simulink model "ICN_with_BR_input_model4test_clusterParams_ICNtune_v13_RSA_25Hz"  (R2020b)
settings: Solver=ode15s  StartTime=0.5  StopTime=300  RelTol=1e-3  EnableMultiTasking=on
model workspace (MAT data in the model file):
  HRResponseIano = [1 0.976355617701 1.05061592575 1.14391807051 1.22959062218 1.30026078221 1.35513299833 1.39551709306 1.423380234 1.44057518669 1.44870724956 1.44945189675 ... (1201 elements, 1x1201)]
values from neighbouring files (symbols this model uses):
  LBNP_input = Simulink.Parameter(LBNP_input)    [BRclosedLoop_model_initialize_params.m]
libraries: simulink x1
(part 1 of 2)
settings Model: OrderedModelArguments=off  Creator=parkjams  LastModifiedBy=mmgee
settings SolverCC: ZeroCrossAlgorithm=Adaptive
settings DataIOCC: SaveFormat=StructureWithTime  ReturnWorkspaceOutputs=off
settings OptimizationCC: LifeSpan=inf
settings DebuggingCC: IgnoredZcDiagnostic=none  SFUnexpectedBacktrackingDiag=warning  SFNoUnconditionalDefaultTransitionDiag=warning  SFExecutionAtInitializationDiag=none  ArithmeticOperatorsInVariantConditions=warning
settings HardwareCC: ProdBitPerSizeT=32  ProdBitPerPtrDiffT=32  ProdWordSize=32  ProdHWDeviceType=Specified  TargetBitPerPointer=64  TargetBitPerSizeT=64  TargetBitPerPtrDiffT=64  TargetLongLongMode=on  TargetIntDivRoundTo=Zero  TargetEndianess=LittleEndian  TargetWordSize=64  TargetHWDeviceType=MATLAB Host  ProdEqTarget=off
settings ModelReferenceCC: PropagateSignalLabelsOutOfModel=off
settings SFSimCC: SimUseLocalCustomCode=off  CustomCodeUndefinedFunction=UseInterfaceOnly
settings RTWCC: Description=Rapid Simulation Target  SystemTargetFile=rsim.tlc  TemplateMakefile=rsim_default_tmf  RTWUseLocalCustomCode=off
settings CodeAppCC: StateflowObjectComments=on
settings ConfigComp: CovMetricSettings=dw  CovSaveCumulativeToWorkspaceVar=on  CovSaveSingleToWorkspaceVar=on  CovExternalEMLEnable=off

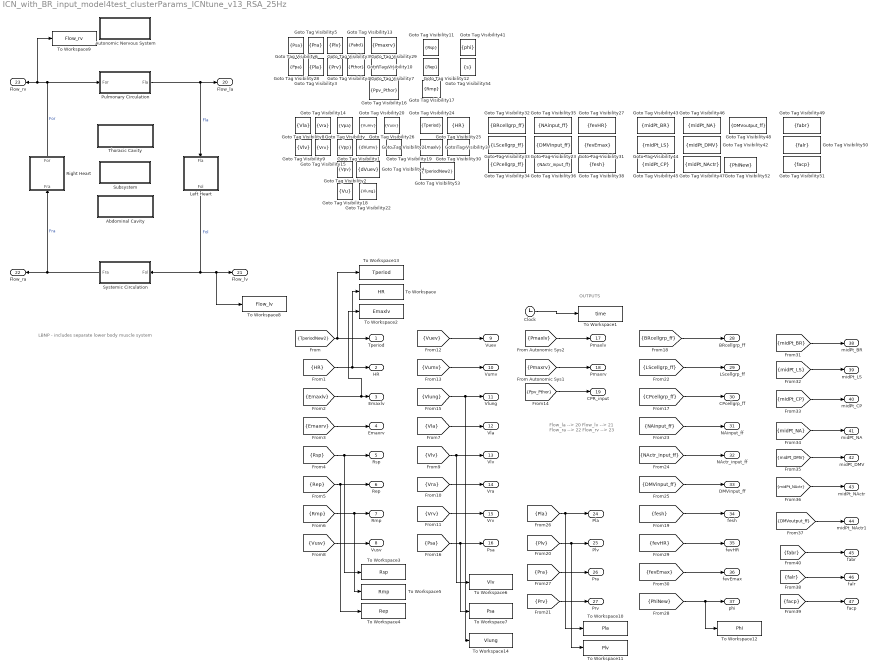
== system ICN_with_BR_input_model4test_clusterParams_ICNtune_v13_RSA_25Hz ==
  note: Flow_la --> 20
      |
      | Flow_lv --> 21
      |
      | Flow_ra --> 22
      |
      | Flow_rv --> 23
  note: OUTPUTS
  note: LBNP - includes separate lower body muscle system
  Abdominal Cavity : Subsystem
      mask Display: disp('Abdominal Cavity')
  Autonomic Nervous System : Subsystem
      mask Display: disp('Autonomic \n Nervous System')
  Clock : Clock
  Goto Tag Visibility : GotoTagVisibility  GotoTag=Vpa
  Goto Tag Visibility1 : GotoTagVisibility  GotoTag=Vpp
  Goto Tag Visibility10 : GotoTagVisibility  GotoTag=Pthor
  Goto Tag Visibility11 : GotoTagVisibility  GotoTag=Rsp
  Goto Tag Visibility12 : GotoTagVisibility  GotoTag=Rep
  Goto Tag Visibility13 : GotoTagVisibility  GotoTag=Pabd
  Goto Tag Visibility14 : GotoTagVisibility  GotoTag=Vra
  Goto Tag Visibility15 : GotoTagVisibility  GotoTag=Vrv
  Goto Tag Visibility16 : GotoTagVisibility  GotoTag=Ppv_Pthor
  Goto Tag Visibility17 : GotoTagVisibility  GotoTag=Rmp
  Goto Tag Visibility18 : GotoTagVisibility  GotoTag=Vu
  Goto Tag Visibility19 : GotoTagVisibility  GotoTag=Vuev
  Goto Tag Visibility2 : GotoTagVisibility  GotoTag=Vpv
  Goto Tag Visibility20 : GotoTagVisibility  GotoTag=Vumv
  Goto Tag Visibility21 : GotoTagVisibility  GotoTag=dVumv
  Goto Tag Visibility22 : GotoTagVisibility  GotoTag=Vlung
  Goto Tag Visibility23 : GotoTagVisibility  GotoTag=DMVinput_ff
  Goto Tag Visibility24 : GotoTagVisibility  GotoTag=Tperiod
  Goto Tag Visibility25 : GotoTagVisibility  GotoTag=HR
  Goto Tag Visibility26 : GotoTagVisibility  GotoTag=Vusv
  Goto Tag Visibility27 : GotoTagVisibility  GotoTag=fevHR
  Goto Tag Visibility28 : GotoTagVisibility  GotoTag=Ppa
  Goto Tag Visibility29 : GotoTagVisibility  GotoTag=Pmaxrv
  Goto Tag Visibility3 : GotoTagVisibility  GotoTag=Pla
  Goto Tag Visibility30 : GotoTagVisibility  GotoTag=Emaxrv
  Goto Tag Visibility31 : GotoTagVisibility  GotoTag=fevEmax
  Goto Tag Visibility32 : GotoTagVisibility  GotoTag=BRcellgrp_ff
  Goto Tag Visibility33 : GotoTagVisibility  GotoTag=LScellgrp_ff
  Goto Tag Visibility34 : GotoTagVisibility  GotoTag=CPcellgrp_ff
  Goto Tag Visibility35 : GotoTagVisibility  GotoTag=NAinput_ff
  Goto Tag Visibility36 : GotoTagVisibility  GotoTag=NActr_input_ff
  Goto Tag Visibility37 : GotoTagVisibility  GotoTag=Emaxlv
  Goto Tag Visibility38 : GotoTagVisibility  GotoTag=fesh
  Goto Tag Visibility39 : GotoTagVisibility  GotoTag=Plv
  Goto Tag Visibility4 : GotoTagVisibility  GotoTag=dVuev
  Goto Tag Visibility40 : GotoTagVisibility  GotoTag=Prv
  Goto Tag Visibility41 : GotoTagVisibility  GotoTag=phi
  Goto Tag Visibility42 : GotoTagVisibility  GotoTag=midPt_DMV
  Goto Tag Visibility43 : GotoTagVisibility  GotoTag=midPt_BR
  Goto Tag Visibility44 : GotoTagVisibility  GotoTag=midPt_LS
  Goto Tag Visibility45 : GotoTagVisibility  GotoTag=midPt_CP
  Goto Tag Visibility46 : GotoTagVisibility  GotoTag=midPt_NA
  Goto Tag Visibility47 : GotoTagVisibility  GotoTag=midPt_NActr
  Goto Tag Visibility48 : GotoTagVisibility  GotoTag=DMVoutput_ff
  Goto Tag Visibility49 : GotoTagVisibility  GotoTag=fabr
  Goto Tag Visibility5 : GotoTagVisibility  GotoTag=Pra
  Goto Tag Visibility50 : GotoTagVisibility  GotoTag=falr
  Goto Tag Visibility51 : GotoTagVisibility  GotoTag=facp
  Goto Tag Visibility52 : GotoTagVisibility  GotoTag=PhiNew
  Goto Tag Visibility53 : GotoTagVisibility  GotoTag=TperiodNew2
  Goto Tag Visibility54 : GotoTagVisibility  GotoTag=s
  Goto Tag Visibility6 : GotoTagVisibility  GotoTag=Psa
  Goto Tag Visibility7 : GotoTagVisibility  GotoTag=Pmaxlv
  Goto Tag Visibility8 : GotoTagVisibility  GotoTag=Vla
  Goto Tag Visibility9 : GotoTagVisibility  GotoTag=Vlv
  Left Heart : Subsystem
      mask Display: disp('Left Heart')
  Pulmonary Circulation : Subsystem
      mask Display: disp('Pulmonary \n Circulation')
  Right Heart : Subsystem
      mask Display: disp('Right Heart')
  Subsystem : Subsystem
      mask Display: disp('Lungs')
  Systemic Circulation : Subsystem
      mask Display: disp('Systemic \n Circulation')
  Thoracic Cavity : Subsystem
      mask Display: disp('Thoracic Cavity')
  To Workspace : ToWorkspace  VariableName=HR  SampleTime=-1
  To Workspace1 : ToWorkspace  VariableName=time  SampleTime=-1
  To Workspace10 : ToWorkspace  VariableName=Pla  SampleTime=-1
  To Workspace11 : ToWorkspace  VariableName=Plv  SampleTime=-1
  To Workspace12 : ToWorkspace  VariableName=Phi  SampleTime=-1
  To Workspace13 : ToWorkspace  VariableName=Tperiod  SampleTime=-1
  To Workspace14 : ToWorkspace  VariableName=Vlung  SampleTime=-1
  To Workspace2 : ToWorkspace  VariableName=Emaxlv  SampleTime=-1
  To Workspace3 : ToWorkspace  VariableName=Rsp  SaveFormat=Timeseries  SampleTime=-1
  To Workspace4 : ToWorkspace  VariableName=Rep  SaveFormat=Timeseries  SampleTime=-1
  To Workspace5 : ToWorkspace  VariableName=Rmp  SaveFormat=Timeseries  SampleTime=-1
  To Workspace6 : ToWorkspace  VariableName=Vlv  SampleTime=-1
  To Workspace7 : ToWorkspace  VariableName=Psa  SampleTime=-1
  To Workspace8 : ToWorkspace  VariableName=Flow_lv  SampleTime=-1
  To Workspace9 : ToWorkspace  VariableName=Flow_rv  SampleTime=-1
  Tperiod : Outport
  HR : Outport  Port=2
  Emaxlv : Outport  Port=3
  Emaxrv : Outport  Port=4
  Rsp : Outport  Port=5
  Rep : Outport  Port=6
  Rmp : Outport  Port=7
  Vusv : Outport  Port=8
  Vuev : Outport  Port=9
  Vumv : Outport  Port=10
  Vlung : Outport  Port=11
  Vla : Outport  Port=12
  Vlv : Outport  Port=13
  Vra : Outport  Port=14
  Vrv : Outport  Port=15
  Psa : Outport  Port=16
  Pmaxlv : Outport  Port=17
  Pmaxrv : Outport  Port=18
  CPR_input : Outport  Port=19
  Flow_la : Outport  Port=20
  Flow_lv : Outport  Port=21
  Flow_ra : Outport  Port=22
  Flow_rv : Outport  Port=23
  Pla : Outport  Port=24
  Plv : Outport  Port=25
  Pra : Outport  Port=26
  Prv : Outport  Port=27
  BRcellgrp_ff : Outport  Port=28
  LScellgrp_ff : Outport  Port=29
  CPcellgrp_ff : Outport  Port=30
  NAinput_ff : Outport  Port=31
  NActr_input_ff : Outport  Port=32
  DMVinput_ff : Outport  Port=33
  fesh : Outport  Port=34
  fevHR : Outport  Port=35
  fevEmax : Outport  Port=36
  phi : Outport  Port=37
  midPt_BR : Outport  Port=38
  midPt_LS : Outport  Port=39
  midPt_CP : Outport  Port=40
  midPt_NA : Outport  Port=41
  midPt_DMV : Outport  Port=42
  midPt_NActr : Outport  Port=43
  midPt_NActr1 : Outport  Port=44
  fabr : Outport  Port=45
  falr : Outport  Port=46
  facp : Outport  Port=47
  wires:
  Pulmonary Circulation/1(Fla) -> Left Heart/1(Fla), Flow_la/1  "Fla"
  Right Heart/1(For) -> To Workspace9/1, Flow_rv/1, Pulmonary Circulation/1(For)  "For"
  Left Heart/1(Fol) -> Systemic Circulation/1(Fol), To Workspace8/1, Flow_lv/1  "Fol"
  Systemic Circulation/1(Fra) -> Right Heart/1(Fra), Flow_ra/1  "Fra"
  [TperiodNew2] -> To Workspace13/1, Tperiod/1
  [HR] -> To Workspace/1, HR/1
  [Emaxlv] -> To Workspace2/1, Emaxlv/1
  [Emaxrv] -> Emaxrv/1
  [Rsp] -> To Workspace3/1, Rsp/1
  [Rep] -> To Workspace4/1, Rep/1
  [Rmp] -> To Workspace5/1, Rmp/1
  [Vusv] -> Vusv/1
  [Vuev] -> Vuev/1
  [Vumv] -> Vumv/1
  [Vlung] -> To Workspace14/1, Vlung/1
  [Vla] -> Vla/1
  [Vlv] -> To Workspace6/1, Vlv/1
  [Vra] -> Vra/1
  [Vrv] -> Vrv/1
  [Psa] -> To Workspace7/1, Psa/1
  [Pmaxlv] -> Pmaxlv/1
  [Pmaxrv] -> Pmaxrv/1
  [Ppv_Pthor] -> CPR_input/1
  [Pla] -> To Workspace10/1, Pla/1
  [Plv] -> To Workspace11/1, Plv/1
  [Pra] -> Pra/1
  [Prv] -> Prv/1
  [BRcellgrp_ff] -> BRcellgrp_ff/1
  [LScellgrp_ff] -> LScellgrp_ff/1
  [CPcellgrp_ff] -> CPcellgrp_ff/1
  [NAinput_ff] -> NAinput_ff/1
  [NActr_input_ff] -> NActr_input_ff/1
  [DMVinput_ff] -> DMVinput_ff/1
  [fesh] -> fesh/1
  [fevHR] -> fevHR/1
  [fevEmax] -> fevEmax/1
  [PhiNew] -> To Workspace12/1, phi/1
  [midPt_BR] -> midPt_BR/1
  [midPt_LS] -> midPt_LS/1
  [midPt_CP] -> midPt_CP/1
  [midPt_NA] -> midPt_NA/1
  [midPt_DMV] -> midPt_DMV/1
  [midPt_NActr] -> midPt_NActr/1
  [DMVoutput_ff] -> midPt_NActr1/1
  [fabr] -> fabr/1
  [falr] -> falr/1
  [facp] -> facp/1
  Clock/1 -> To Workspace1/1

== system ICN_with_BR_input_model4test_clusterParams_ICNtune_v13_RSA_25Hz/Abdominal Cavity ==
  (Tinsp + Texp)/Tresp : Switch  Criteria=u2 > Threshold  Threshold=(1.6 + 1.4)/4
  Abdominal condition 1 : Subsystem
  Abdominal condition 2 : Subsystem
  Constant : Constant  Value=-2.5
  Constant2 : Constant  Value=0
  Integral threshold : Constant
  Integrator3 : Integrator  ExternalReset=falling  ShowStatePort=on
  Math Function3 : Math  Operator=reciprocal  SignedPower=on  SaturateOnIntegerOverflow=on
  Sum3 : Sum  Inputs=-+
  Tinsp/(2*Tresp) : Switch  Criteria=u2 > Threshold  Threshold=1.6/(2*4)
  Tinsp/Tresp : Switch  Criteria=u2 > Threshold  Threshold=1.6/4
  Tresp : Constant  Value=4
  tag scope: Pabd=scoped
  wires:
  Tresp/1 -> Math Function3/1
  Math Function3/1 -> Integrator3/1
  Integrator3/State -> Sum3/1
  Integral threshold/1 -> Sum3/2
  Sum3/1 -> Integrator3/2
  Integrator3/1 -> Abdominal condition 1/1(S (resp)), (Tinsp + Texp)/Tresp/2, Abdominal condition 2/1(S (resp)), Tinsp/Tresp/2, Tinsp/(2*Tresp)/2
  Abdominal condition 1/1(Out1) -> Tinsp/(2*Tresp)/3
  Constant/1 -> Tinsp/(2*Tresp)/1
  Tinsp/(2*Tresp)/1 -> Tinsp/Tresp/3
  Abdominal condition 2/1(Out1) -> Tinsp/Tresp/1
  Tinsp/Tresp/1 -> (Tinsp + Texp)/Tresp/3
  Constant2/1 -> (Tinsp + Texp)/Tresp/1
  (Tinsp + Texp)/Tresp/1 -> [Pabd]

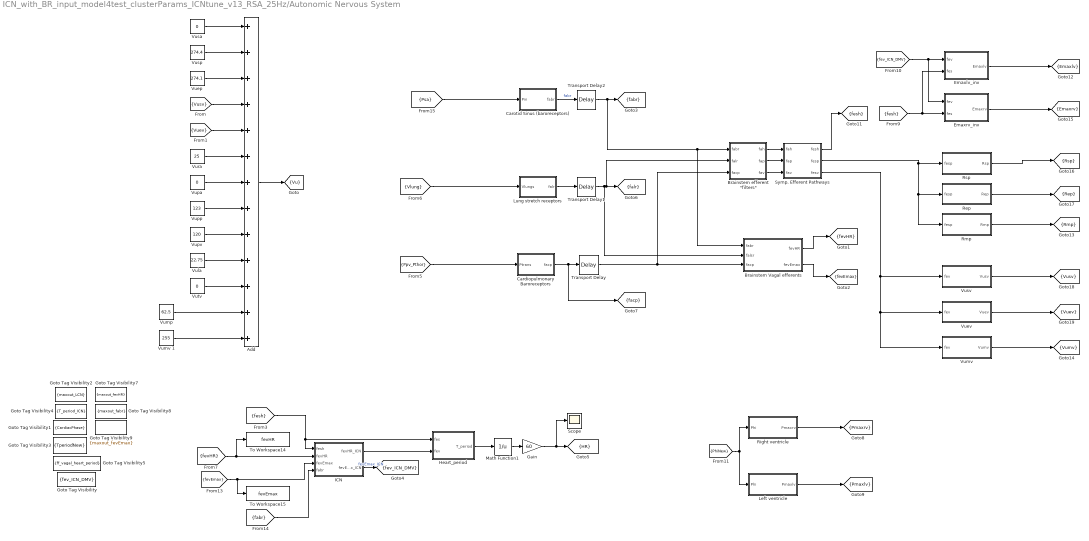
== system ICN_with_BR_input_model4test_clusterParams_ICNtune_v13_RSA_25Hz/Autonomic Nervous System ==
  " Brainstem efferent \"filters\"" : Subsystem
  " Symp. Efferent Pathways" : Subsystem
  Add : Sum  Inputs=+++++++++++++
  "Brainstem Vagal efferents " : Subsystem
  Cardiopulmonary Baroreceptors : Subsystem
  Carotid Sinus (baroreceptors) : Subsystem
  Emaxlv_inv : Subsystem
  Emaxrv_inv : Subsystem
  Gain : Gain  Gain=60
  Goto Tag Visibility : GotoTagVisibility  GotoTag=fev_ICN_DMV
  Goto Tag Visibility1 : GotoTagVisibility  GotoTag=CardiacPhase
  Goto Tag Visibility2 : GotoTagVisibility  GotoTag=maxout_LCN
  Goto Tag Visibility3 : GotoTagVisibility  GotoTag=TperiodNew
  Goto Tag Visibility4 : GotoTagVisibility  GotoTag=T_period_ICN
  Goto Tag Visibility5 : GotoTagVisibility  GotoTag=ff_vagal_heart_period
  Goto Tag Visibility7 : GotoTagVisibility  GotoTag=maxout_fevHR
  Goto Tag Visibility8 : GotoTagVisibility  GotoTag=maxout_fabr
  Goto Tag Visibility9 : GotoTagVisibility  GotoTag=maxout_fevEmax
  Heart_period : Subsystem
  ICN : Subsystem
  Left ventricle : Subsystem
  Lung stretch receptors : Subsystem
  Math Function1 : Math  Operator=reciprocal  SignedPower=on  SaturateOnIntegerOverflow=on
  Rep : Subsystem
  Right ventricle : Subsystem
  Rmp : Subsystem
  Rsp : Subsystem
  Scope : Scope
  To Workspace14 : ToWorkspace  VariableName=fevHR  SampleTime=-1
  To Workspace15 : ToWorkspace  VariableName=fevEmax  SampleTime=-1
  Transport Delay : TransportDelay  DelayTime=0.03
  Transport Delay1 : TransportDelay  DelayTime=0.03
  Transport Delay2 : TransportDelay  DelayTime=0.03
  Vuep : Constant  Value=274.1
  Vuev : Subsystem
  Vula : Constant  Value=22.75
  Vump : Constant  Value=62.5
  Vumv : Subsystem
  Vumv 1 : Constant  Value=255
  Vupa : Constant  Value=0
  Vupp : Constant  Value=123
  Vupv : Constant  Value=120
  Vura : Constant  Value=25
  Vusa : Constant  Value=0
  Vusp : Constant  Value=274.4
  Vusv : Subsystem
  Vutv : Constant  Value=0
  tag scope: Emaxlv=scoped, Emaxrv=scoped, HR=scoped, Pmaxlv=scoped, Pmaxrv=scoped, Rep=scoped, Rmp=scoped, Rsp=scoped, Vu=scoped, Vuev=scoped, Vumv=scoped, Vusv=scoped, fabr=scoped, facp=scoped, falr=scoped, fesh=scoped, fevEmax=scoped, fevHR=scoped, fev_ICN_DMV=scoped
  wires:
  Vusa/1 -> Add/1
  Vusp/1 -> Add/2
  [Vusv] -> Add/4
  [Vuev] -> Add/5
  Vuep/1 -> Add/3
  Vura/1 -> Add/6
  Vupa/1 -> Add/7
  Vupp/1 -> Add/8
  Vupv/1 -> Add/9
  Vula/1 -> Add/10
  Add/1 -> [Vu]
  Carotid Sinus (baroreceptors)/1(fabr) -> Transport Delay2/1  "fabr"
  Right ventricle/1(Pmaxrv) -> [Pmaxrv]
  Left ventricle/1(Pmaxlv) -> [Pmaxlv]
  Gain/1 -> Scope/1, [HR]
  Math Function1/1 -> Gain/1
  Rsp/1(Rsp) -> [Rsp]
  Rep/1(Rep) -> [Rep]
  Vusv/1(Vusv) -> [Vusv]
  Vuev/1(Vuev) -> [Vuev]
  Vumv/1(Vumv) -> [Vumv]
  Rmp/1(Rmp) -> [Rmp]
  Vump/1 -> Add/12
  Vumv 1/1 -> Add/13
  Lung stretch receptors/1(falr) -> Transport Delay1/1
  Vutv/1 -> Add/11
  [fesh] -> Emaxrv_inv/2(fes), Emaxlv_inv/2(fes)
  "Brainstem Vagal efferents "/2(fevEmax) -> [fevEmax]
  "Brainstem Vagal efferents "/1(fevHR) -> [fevHR]
  Emaxlv_inv/1(Emaxlv) -> [Emaxlv]
  Emaxrv_inv/1(Emaxrv) -> [Emaxrv]
  Cardiopulmonary Baroreceptors/1(facp) -> Transport Delay/1, [facp]
  " Brainstem efferent \"filters\""/1(fah) -> " Symp. Efferent Pathways"/1(fah)
  " Brainstem efferent \"filters\""/2(fap) -> " Symp. Efferent Pathways"/2(fap)
  " Symp. Efferent Pathways"/1(fesh) -> [fesh]
  " Symp. Efferent Pathways"/2(fesp) -> Rmp/1(fesp), Rep/1(fesp), Rsp/1(fesp)
  " Brainstem efferent \"filters\""/3(fav) -> " Symp. Efferent Pathways"/3(fav)
  " Symp. Efferent Pathways"/3(fesv) -> Vumv/1(fev), Vuev/1(fev), Vusv/1(fev)
  [fev_ICN_DMV] -> Emaxrv_inv/1(fev), Emaxlv_inv/1(fev)
  ICN/1(fevHR_ICN) -> Heart_period/2(fev)
  [PhiNew] -> Left ventricle/1(Phi), Right ventricle/1(Phi)
  Heart_period/1(T_period) -> Math Function1/1
  [fesh] -> ICN/1(fesh), Heart_period/1(fes)
  [fevEmax] -> ICN/3(fevEmax), To Workspace15/1
  [fabr] -> ICN/4(fabr)
  [fevHR] -> ICN/2(fevHR), To Workspace14/1
  [Vlung] -> Lung stretch receptors/1(Vlungs)
  [Psa] -> Carotid Sinus (baroreceptors)/1(Pin)
  Transport Delay/1 -> " Brainstem efferent \"filters\""/3(facp), "Brainstem Vagal efferents "/3(facp)
  Transport Delay1/1 -> "Brainstem Vagal efferents "/2(falsr), [falr], " Brainstem efferent \"filters\""/2(falr)
  Transport Delay2/1 -> "Brainstem Vagal efferents "/1(fabr), " Brainstem efferent \"filters\""/1(fabr), [fabr]
  [Ppv_Pthor] -> Cardiopulmonary Baroreceptors/1(Ptrans)
  ICN/2(fevEmax_ICN) -> [fev_ICN_DMV]  "fevEmax_ICN"

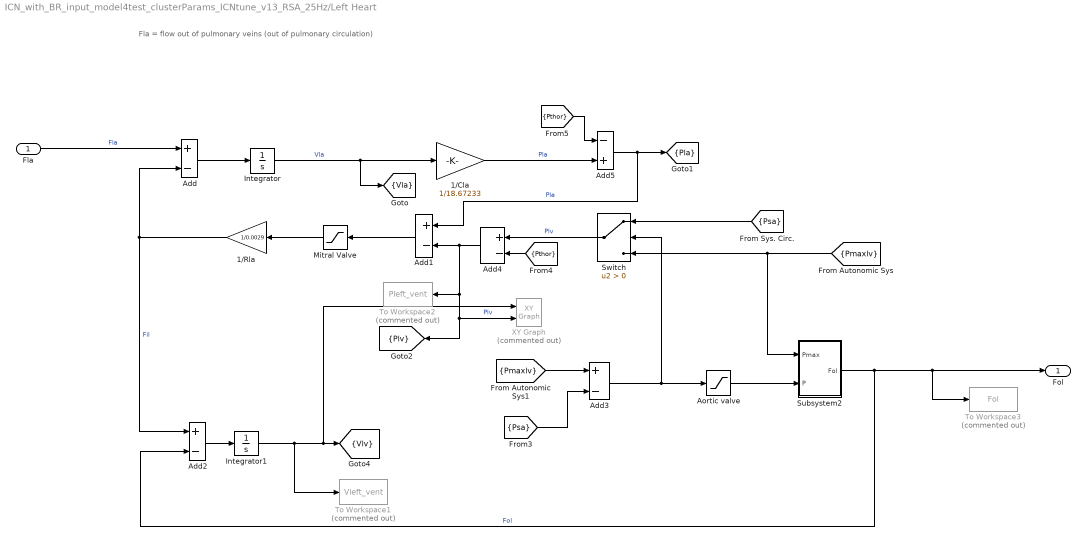
== system ICN_with_BR_input_model4test_clusterParams_ICNtune_v13_RSA_25Hz/Left Heart ==
  note: Fla = flow out of pulmonary veins (out of pulmonary circulation)
  Fla : Inport
  1/Cla : Gain  Gain=1/18.67233
  1/Rla : Gain  Gain=1/0.0029
  Add{,1..4} (5 alike) : Sum  Inputs=+-
  Add5 : Sum  Inputs=-+
  Aortic valve : Saturate  UpperLimit=inf  LowerLimit=0
  Integrator : Integrator
  Integrator1 : Integrator
  Mitral Valve : Saturate  UpperLimit=inf  LowerLimit=0
  Subsystem2 : Subsystem
  Switch : Switch  Criteria=u2 > Threshold
  To Workspace1 : ToWorkspace  Commented=on  VariableName=Vleft_vent  SaveFormat=Timeseries  SampleTime=-1
  To Workspace2 : ToWorkspace  Commented=on  VariableName=Pleft_vent  SaveFormat=Timeseries  SampleTime=-1
  To Workspace3 : ToWorkspace  Commented=on  VariableName=Fol  SaveFormat=Timeseries  SampleTime=-1
  XY Graph : simulink/Sinks/XY Graph  Commented=on  xmin=0  xmax=200  ymin=0  ymax=150  st=-1
  Fol : Outport
  tag scope: Pla=scoped, Plv=scoped, Vla=scoped, Vlv=scoped
  wires:
  Add/1 -> Integrator/1
  [Psa] -> Switch/1
  [Pmaxlv] -> Subsystem2/1(Pmax), Switch/3
  [Pmaxlv] -> Add3/1
  [Psa] -> Add3/2
  Add3/1 -> Switch/2, Aortic valve/1
  Add1/1 -> Mitral Valve/1
  Mitral Valve/1 -> 1/Rla/1
  1/Rla/1 -> Add/2, Add2/1  "Fil"
  Aortic valve/1 -> Subsystem2/2(P)
  Subsystem2/1(Fol) -> Add2/2, To Workspace3/1, Fol/1  "Fol"
  Add2/1 -> Integrator1/1
  Integrator1/1 -> To Workspace1/1, XY Graph/1, [Vlv]
  Fla/1 -> Add/1  "Fla"
  Integrator/1 -> 1/Cla/1, [Vla]  "Vla"
  1/Cla/1 -> Add5/2  "Pla"
  Add5/1 -> Add1/1, [Pla]  "Pla"
  Add4/1 -> XY Graph/2, [Plv], To Workspace2/1, Add1/2  "Plv"
  Switch/1 -> Add4/1  "Plv"
  [Pthor] -> Add4/2
  [Pthor] -> Add5/1

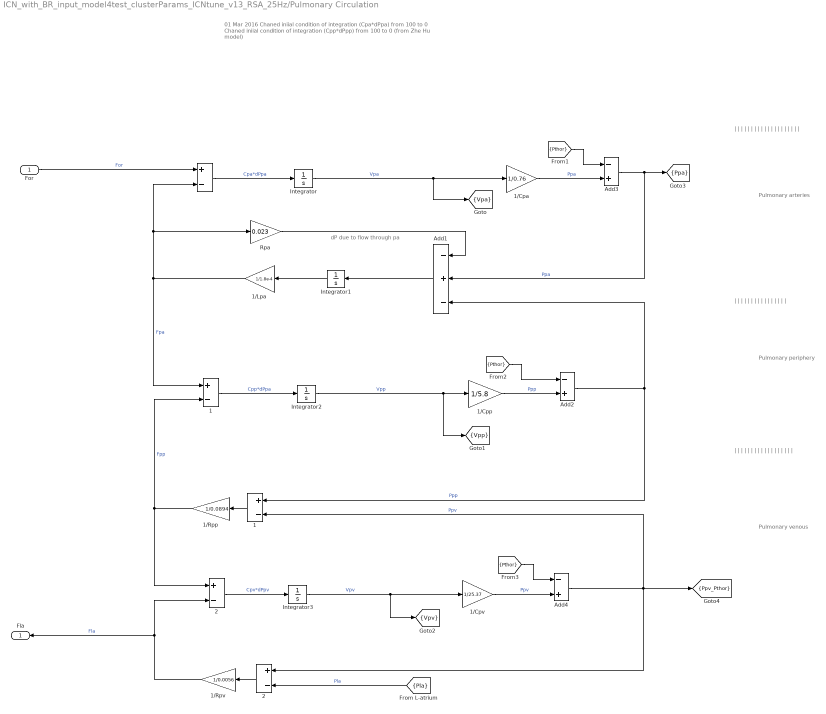
== system ICN_with_BR_input_model4test_clusterParams_ICNtune_v13_RSA_25Hz/Pulmonary Circulation ==
  note: 01 Mar 2016
      | Chaned iniial condition of integration (Cpa*dPpa) from 100 to 0
      | Chaned iniial condition of integration (Cpp*dPpp) from 100 to 0
      | (from Zhe Hu model)
  note: Pulmonary arteries
  note: |
      |         |
      |         |
      |         |
      |         |
      |         |
      |         |
      |         |
      |         |
      |         |
      |         |
      |         |
      |         |
      |         |
      |         |
      |         |
      |         |
      |         |
      |         |
      |         |
  note: dP due to flow through pa
  note: |
      |         |
      |         |
      |         |
      |         |
      |         |
      |         |
      |         |
      |         |
      |         |
      |         |
      |         |
      |         |
      |         |
      |         |
      |         |
  note: |
      |         |
      |         |
      |         |
      |         |
      |         |
      |         |
      |         |
      |         |
      |         |
      |         |
      |         |
      |         |
      |         |
      |         |
      |         |
      |         |
      |         |
  note: Pulmonary periphery
  note: Pulmonary venous
  For : Inport
  " 1" : Sum  Inputs=+-
  "    " : Sum  Inputs=+-
  "   1/Lpa" : Gain  Gain=1/1.8e-4
  "  2" : Sum  Inputs=+-
  1 : Sum  Inputs=+-
  1/Cpa : Gain  Gain=1/0.76
  1/Cpp : Gain  Gain=1/5.8
  1/Cpv : Gain  Gain=1/25.37
  "1/Rpp " : Gain  Gain=1/0.0894
  1/Rpv : Gain  Gain=1/0.0056
  2 : Sum  Inputs=+-
  Add1 : Sum  Inputs=-+-
  Add2 : Sum  Inputs=-+
  Add3 : Sum  Inputs=-+
  Add4 : Sum  Inputs=-+
  Integrator : Integrator  InitialCondition=100
  Integrator1 : Integrator
  Integrator2 : Integrator  InitialCondition=100
  Integrator3 : Integrator
  "Rpa " : Gain  Gain=0.023
  Fla : Outport
  tag scope: Ppa=scoped, Ppv_Pthor=scoped, Vpa=scoped, Vpp=scoped, Vpv=scoped
  wires:
  Add1/1 -> Integrator1/1
  [Pla] -> "  2"/2  "Pla"
  Integrator1/1 -> "   1/Lpa"/1
  "   1/Lpa"/1 -> 1/1, "Rpa "/1, "    "/2  "Fpa"
  "1/Rpp "/1 -> 1/2, 2/1  "Fpp"
  " 1"/1 -> "1/Rpp "/1
  "    "/1 -> Integrator/1  "Cpa*dPpa"
  1/1 -> Integrator2/1  "Cpp*dPpa"
  2/1 -> Integrator3/1  "Cpv*dPpv"
  1/Rpv/1 -> 2/2, Fla/1  "Fla"
  "  2"/1 -> 1/Rpv/1
  For/1 -> "    "/1  "For"
  1/Cpa/1 -> Add3/2  "Ppa"
  [Pthor] -> Add3/1
  Add3/1 -> Add1/2, [Ppa]  "Ppa"
  [Pthor] -> Add2/1
  1/Cpp/1 -> Add2/2  "Ppp"
  Add2/1 -> Add1/3, " 1"/1  "Ppp"
  [Pthor] -> Add4/1
  1/Cpv/1 -> Add4/2  "Ppv"
  Add4/1 -> "  2"/1, [Ppv_Pthor], " 1"/2  "Ppv"
  Integrator/1 -> [Vpa], 1/Cpa/1  "Vpa"
  Integrator2/1 -> [Vpp], 1/Cpp/1  "Vpp"
  Integrator3/1 -> 1/Cpv/1, [Vpv]  "Vpv"
  "Rpa "/1 -> Add1/1

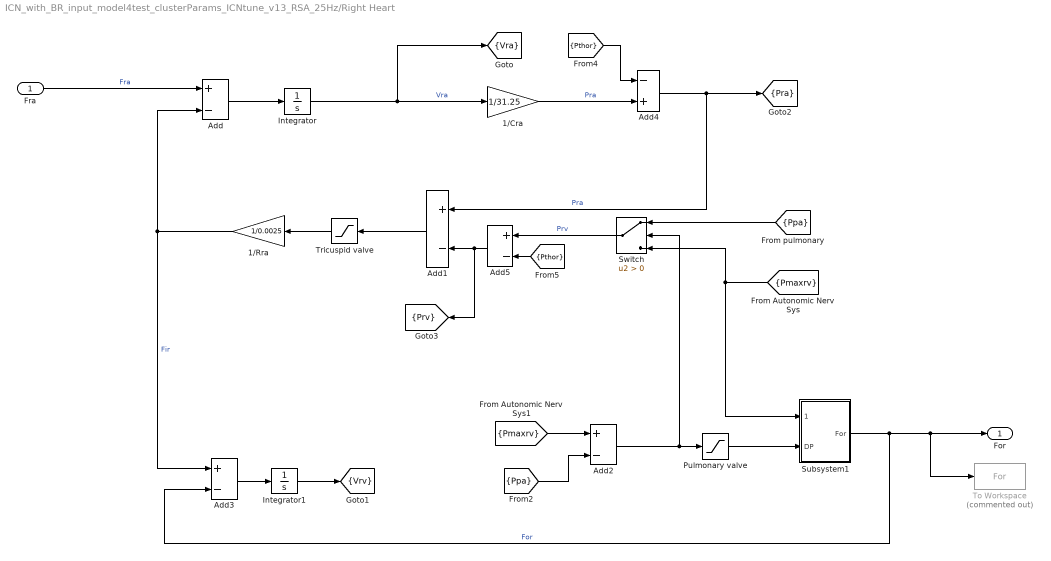
== system ICN_with_BR_input_model4test_clusterParams_ICNtune_v13_RSA_25Hz/Right Heart ==
  Fra : Inport
  1/Cra : Gain  Gain=1/31.25
  1/Rra : Gain  Gain=1/0.0025
  Add{,1..3,5} (5 alike) : Sum  Inputs=+-
  Add4 : Sum  Inputs=-+
  Integrator : Integrator
  Integrator1 : Integrator
  Pulmonary valve : Saturate  UpperLimit=inf  LowerLimit=0
  Subsystem1 : Subsystem
  Switch : Switch  Criteria=u2 > Threshold
  To Workspace : ToWorkspace  Commented=on  VariableName=For  SaveFormat=Timeseries  SampleTime=-1
  Tricuspid valve : Saturate  UpperLimit=inf  LowerLimit=0  ZeroCross=off
  For : Outport
  tag scope: Pra=scoped, Prv=scoped, Vra=scoped, Vrv=scoped
  wires:
  1/Rra/1 -> Add/2, Add3/1  "Fir"
  [Ppa] -> Switch/1
  [Pmaxrv] -> Switch/3, Subsystem1/1(Pmaxrv)
  [Pmaxrv] -> Add2/1
  [Ppa] -> Add2/2
  Add2/1 -> Pulmonary valve/1, Switch/2
  Pulmonary valve/1 -> Subsystem1/2(DP)
  Subsystem1/1(For) -> Add3/2, To Workspace/1, For/1  "For"
  Add1/1 -> Tricuspid valve/1
  Tricuspid valve/1 -> 1/Rra/1
  Add3/1 -> Integrator1/1
  Fra/1 -> Add/1  "Fra"
  Integrator/1 -> [Vra], 1/Cra/1  "Vra"
  Integrator1/1 -> [Vrv]
  1/Cra/1 -> Add4/2  "Pra"
  Add4/1 -> Add1/1, [Pra]  "Pra"
  Add5/1 -> [Prv], Add1/2
  Switch/1 -> Add5/1  "Prv"
  [Pthor] -> Add4/1
  [Pthor] -> Add5/2
  Add/1 -> Integrator/1

== system ICN_with_BR_input_model4test_clusterParams_ICNtune_v13_RSA_25Hz/Subsystem ==
  Add : Sum  Inputs=+-
  Add1 : Sum  Inputs=+-
  Product : Product
  Vl0 : Constant  Value=1.9
  Vln : Constant  Value=2.3
  alpha : Constant  Value=0.1
  tag scope: Vlung=scoped
  wires:
  Vl0/1 -> Add/1
  alpha/1 -> Product/1
  [Pthor] -> Product/2
  Product/1 -> Add/2
  Add/1 -> Add1/1  "Vl"
  Add1/1 -> [Vlung]
  Vln/1 -> Add1/2  "Vln"

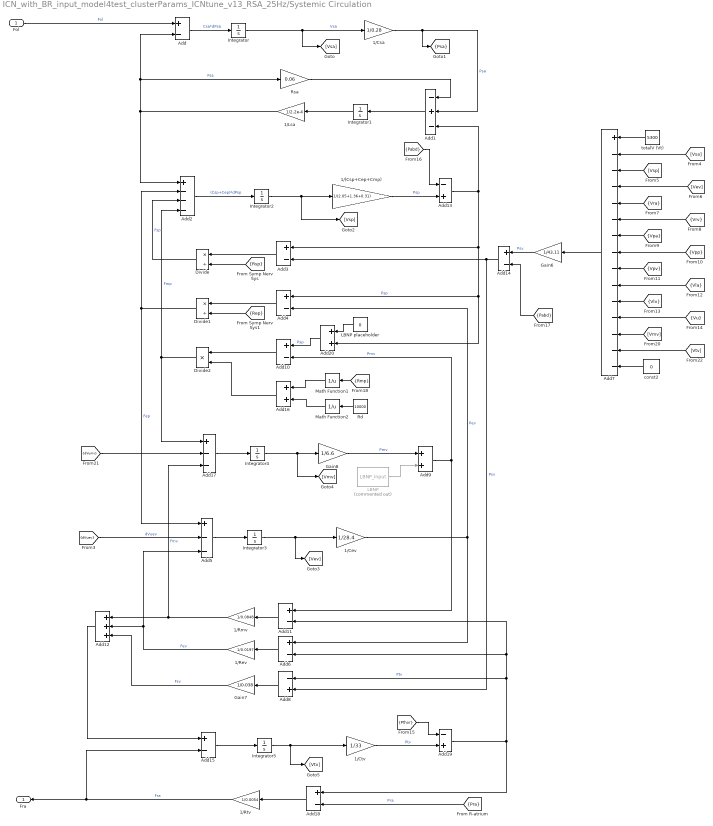
== system ICN_with_BR_input_model4test_clusterParams_ICNtune_v13_RSA_25Hz/Systemic Circulation ==
  Fol : Inport
  1/(Csp+Cep+Cmp) : Gain  Gain=1/(2.05+1.36+0.31)
  1/Cev : Gain  Gain=1/28.4
  1/Csa : Gain  Gain=1/0.28
  1/Ctv : Gain  Gain=1/33
  1/Lsa : Gain  Gain=1/2.2e-4
  1/Rev : Gain  Gain=1/0.0197
  1/Rmv : Gain  Gain=1/0.0848
  1/Rtv : Gain  Gain=1/0.0054
  Add{,3..4,6,10..11,14..15,18} (9 alike) : Sum  Inputs=+-
  Add1 : Sum  Inputs=-+-
  Add12 : Sum  Inputs=+++
  Add13 : Sum  Inputs=-+
  Add16 : Sum
  Add17 : Sum  Inputs=+--
  Add19 : Sum  Inputs=-+
  Add2 : Sum  Inputs=+---
  Add20 : Sum
  Add5 : Sum  Inputs=+--
  Add7 : Sum  Inputs=+--------------
  Add8 : Sum  Inputs=-+
  Add9 : Sum
  Divide : Product  Inputs=*/
  Divide1 : Product  Inputs=*/
  Divide2 : Product  Inputs=**
  Gain6 : Gain  Gain=1/43.11
  Gain7 : Gain  Gain=1/0.038
  Gain8 : Gain  Gain=1/6.6
  Integrator{,1..5} (6 alike) : Integrator
  LBNP : Constant  Commented=on  Value=LBNP_input
  LBNP placeholder : Constant  Value=0
  Math Function1 : Math  Operator=reciprocal  SignedPower=on  SaturateOnIntegerOverflow=on
  Math Function2 : Math  Operator=reciprocal  SignedPower=on  SaturateOnIntegerOverflow=on
  Rd : Constant  Value=10000
  Rsa : Gain  Gain=0.06
  const2 : Constant  Value=0
  totalV (Vt) : Constant  Value=5300
  Fra : Outport
  tag scope: Psa=scoped
  wires:
  Add/1 -> Integrator/1  "Csa*dPsa"
  Add1/1 -> Integrator1/1
  Integrator1/1 -> 1/Lsa/1
  1/Lsa/1 -> Add2/1, Rsa/1, Add/2  "Fsa"
  Add3/1 -> Divide/1
  [Rsp] -> Divide/2
  Divide/1 -> Add2/3  "Fsp"
  Add4/1 -> Divide1/1
  Divide1/1 -> Add5/1, Add2/2  "Fep"
  [Rep] -> Divide1/2
  Add2/1 -> Integrator2/1  "(Csp+Cep)*dPsp"
  Integrator2/1 -> 1/(Csp+Cep+Cmp)/1, [Vsp]
  Add6/1 -> 1/Rev/1
  1/Rev/1 -> Add12/2, Add5/3  "Fev"
  1/Cev/1 -> Add6/1, Add4/2  "Pev"
  [Vsa] -> Add7/2
  [Vev] -> Add7/4
  [Vra] -> Add7/5
  [Vrv] -> Add7/6
  [Vpa] -> Add7/7
  [Vpp] -> Add7/8
  [Vla] -> Add7/10
  [Vlv] -> Add7/11
  [Vu] -> Add7/12
  Add8/1 -> Gain7/1
  Add5/1 -> Integrator3/1
  [dVuev] -> Add5/2  "dVuev"
  Fol/1 -> Add/1  "Fol"
  Add7/1 -> Gain6/1
  [Vsp] -> Add7/3
  [Vpv] -> Add7/9
  Integrator/1 -> 1/Csa/1, [Vsa]  "Vsa"
  Gain7/1 -> Add12/3  "Fsv"
  1/Csa/1 -> [Psa], Add1/2  "Psa"
  [Pabd] -> Add13/1
  1/(Csp+Cep+Cmp)/1 -> Add13/2  "Psp"
  Add13/1 -> Add3/1, Add20/2, Add4/1, Add1/3  "Psp"
  Add14/1 -> Add3/2, Add8/2  "Psv"
  [Pabd] -> Add14/2
  [Rmp] -> Math Function1/1
  Rd/1 -> Math Function2/1
  Math Function1/1 -> Add16/1
  Math Function2/1 -> Add16/2
  Add16/1 -> Divide2/2
  Add10/1 -> Divide2/1
  Divide2/1 -> Add2/4, Add17/1  "Fmp"
  [dVumv] -> Add17/2
  Add17/1 -> Integrator4/1
  Gain8/1 -> Add9/1  "Pmv"
  Add11/1 -> 1/Rmv/1
  1/Rmv/1 -> Add17/3, Add12/1  "Fmv"
  Add15/1 -> Integrator5/1
  1/Ctv/1 -> Add19/2  "Ptv"
  1/Rtv/1 -> Fra/1, Add15/2  "Fra"
  Add19/1 -> Add18/1, Add8/1, Add11/2, Add6/2  "Ptv"
  Add18/1 -> 1/Rtv/1
  [Pthor] -> Add19/1
  Add12/1 -> Add15/1
  [Pra] -> Add18/2  "Pra"
  [Vmv] -> Add7/13
  [Vtv] -> Add7/14
  Integrator4/1 -> [Vmv], Gain8/1
  Integrator3/1 -> 1/Cev/1, [Vev]
  Integrator5/1 -> 1/Ctv/1, [Vtv]
  Add9/1 -> Add11/1, Add10/2  "Pmv"
  LBNP/1 -> Add9/2
  Add20/1 -> Add10/1  "Psp"
  totalV (Vt)/1 -> Add7/1
  Gain6/1 -> Add14/1  "Psv"
  const2/1 -> Add7/15
  Rsa/1 -> Add1/1
  LBNP placeholder/1 -> Add20/1

== system ICN_with_BR_input_model4test_clusterParams_ICNtune_v13_RSA_25Hz/Thoracic Cavity ==
  1 + (Texp/Tinsp) : Switch  Criteria=u2 > Threshold  Threshold=1 + (1.4/1.6)
  Divide2 : Product  Inputs=/*
  Integral threshold : Constant
  Integrator2 : Integrator  ExternalReset=falling  ShowStatePort=on
  Math Function2 : Math  Operator=reciprocal  SignedPower=on  SaturateOnIntegerOverflow=on
  Product4 : Product
  PthorMax1 : Constant  Value=-4
  Sum2 : Sum  Inputs=-+
  Switch4 : Switch  Criteria=u2 > Threshold  Threshold=1
  Thoracic cond. 1 : Subsystem
  Thoracic cond. 2 : Subsystem
  Tinsp : Constant  Value=1.6
  To Workspace : ToWorkspace  Commented=on  VariableName=Pthor  SaveFormat=Timeseries  SampleTime=-1
  Tresp2 : Constant  Value=4
  tag scope: Pthor=scoped, s=scoped
  wires:
  Tresp2/1 -> Divide2/2, Math Function2/1
  Math Function2/1 -> Integrator2/1
  Integrator2/State -> Sum2/1
  Integral threshold/1 -> Sum2/2
  Sum2/1 -> Integrator2/2
  Integrator2/1 -> Thoracic cond. 2/1(S (resp)), Product4/2, Thoracic cond. 1/1(S (resp)), [s]  "S"
  Tinsp/1 -> Divide2/1
  Divide2/1 -> Product4/1
  Product4/1 -> 1 + (Texp/Tinsp)/2, Switch4/2
  Thoracic cond. 2/1(Out1) -> Switch4/1
  Thoracic cond. 1/1(Out1) -> Switch4/3
  Switch4/1 -> 1 + (Texp/Tinsp)/3
  PthorMax1/1 -> 1 + (Texp/Tinsp)/1
  1 + (Texp/Tinsp)/1 -> [Pthor], To Workspace/1

== system ICN_with_BR_input_model4test_clusterParams_ICNtune_v13_RSA_25Hz/Abdominal Cavity/Abdominal condition 1 ==
  S (resp) : Inport
  Constant : Constant  Value=-2.5
  Divide : Product  Inputs=*/
  Gain : Gain  Gain=1/2
  Product : Product  Inputs=3
  Tinsp : Constant  Value=1.6
  Tresp2 : Constant  Value=4
  Out1 : Outport
  wires:
  Tinsp/1 -> Gain/1
  Gain/1 -> Divide/2
  Tresp2/1 -> Divide/1
  Divide/1 -> Product/3
  Constant/1 -> Product/2
  S (resp)/1 -> Product/1
  Product/1 -> Out1/1

== system ICN_with_BR_input_model4test_clusterParams_ICNtune_v13_RSA_25Hz/Abdominal Cavity/Abdominal condition 2 ==
  S (resp) : Inport
  Add : Sum  Inputs=-++
  Constant : Constant  Value=-2.5
  Divide1 : Product  Inputs=*/*
  Product : Product
  Texp : Constant  Value=1.4
  Tinsp : Constant  Value=1.6
  Tresp1 : Constant  Value=4
  Out1 : Outport
  wires:
  Tresp1/1 -> Product/2
  S (resp)/1 -> Product/1
  Product/1 -> Add/1
  Texp/1 -> Add/3, Divide1/2
  Tinsp/1 -> Add/2
  Add/1 -> Divide1/1
  Constant/1 -> Divide1/3
  Divide1/1 -> Out1/1

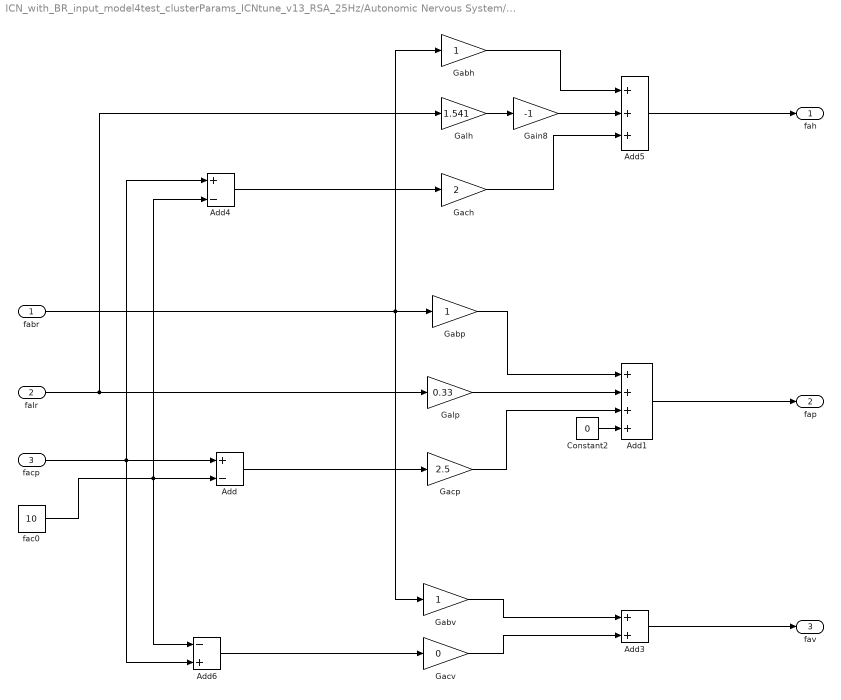
== system ICN_with_BR_input_model4test_clusterParams_ICNtune_v13_RSA_25Hz/Autonomic Nervous System/ Brainstem efferent "filters" ==
  fabr : Inport
  falr : Inport  Port=2
  facp : Inport  Port=3
  Add : Sum  Inputs=+-
  Add1 : Sum  Inputs=++++
  Add3 : Sum
  Add4 : Sum  Inputs=+-
  Add5 : Sum  Inputs=+++
  Add6 : Sum  Inputs=-+
  Constant2 : Constant  Value=0
  Gabh : Gain
  Gabp : Gain
  Gabv : Gain
  Gach : Gain  Gain=2
  Gacp : Gain  Gain=2.5
  Gacv : Gain  Gain=0
  Gain8 : Gain  Gain=-1
  Galh : Gain  Gain=1.541
  Galp : Gain  Gain=0.33
  fac0 : Constant  Value=10
  fah : Outport
  fap : Outport  Port=2
  fav : Outport  Port=3
  wires:
  Gabp/1 -> Add1/1
  Gabv/1 -> Add3/1
  Gacv/1 -> Add3/2
  fac0/1 -> Add4/2, Add6/1, Add/2
  fabr/1 -> Gabv/1, Gabh/1, Gabp/1
  Gabh/1 -> Add5/1
  Gach/1 -> Add5/3
  Add5/1 -> fah/1
  Add4/1 -> Gach/1
  Add/1 -> Gacp/1
  Add6/1 -> Gacv/1
  Gacp/1 -> Add1/3
  facp/1 -> Add4/1, Add6/2, Add/1
  falr/1 -> Galh/1, Galp/1
  Galp/1 -> Add1/2
  Galh/1 -> Gain8/1
  Gain8/1 -> Add5/2
  Add1/1 -> fap/1
  Add3/1 -> fav/1
  Constant2/1 -> Add1/4

== system ICN_with_BR_input_model4test_clusterParams_ICNtune_v13_RSA_25Hz/Autonomic Nervous System/ Symp. Efferent Pathways ==
  fah : Inport
  fap : Inport  Port=2
  fav : Inport  Port=3
  -kes : Gain  Gain=-0.0675
  -kes1 : Gain  Gain=-0.0675
  -kes2 : Gain  Gain=-0.0675
  Add1 : Sum  Inputs=+++
  Add2 : Sum  Inputs=+++
  Add3 : Sum  Inputs=+++
  Math Function1 : Math  SignedPower=on  SaturateOnIntegerOverflow=on
  Math Function2 : Math  SignedPower=on  SaturateOnIntegerOverflow=on
  Math Function3 : Math  SignedPower=on  SaturateOnIntegerOverflow=on
  fes0-fes_inf : Gain  Gain=12.918
  fes0-fes_inf1 : Gain  Gain=12.918
  fes0-fes_inf2 : Gain  Gain=12.918
  fes_cc : Constant  Value=0
  fes_inf : Constant  Value=3.192
  fesh : Outport
  fesp : Outport  Port=2
  fesv : Outport  Port=3
  wires:
  fah/1 -> -kes/1
  Math Function1/1 -> fes0-fes_inf2/1
  fes0-fes_inf2/1 -> Add1/3
  -kes/1 -> Math Function1/1
  fap/1 -> -kes1/1
  Math Function2/1 -> fes0-fes_inf1/1
  -kes1/1 -> Math Function2/1
  fav/1 -> -kes2/1
  Math Function3/1 -> fes0-fes_inf/1
  -kes2/1 -> Math Function3/1
  fes_inf/1 -> Add2/2, Add3/2, Add1/2
  fes_cc/1 -> Add2/1, Add3/1, Add1/1
  fes0-fes_inf1/1 -> Add2/3
  fes0-fes_inf/1 -> Add3/3
  Add1/1 -> fesh/1
  Add2/1 -> fesp/1
  Add3/1 -> fesv/1

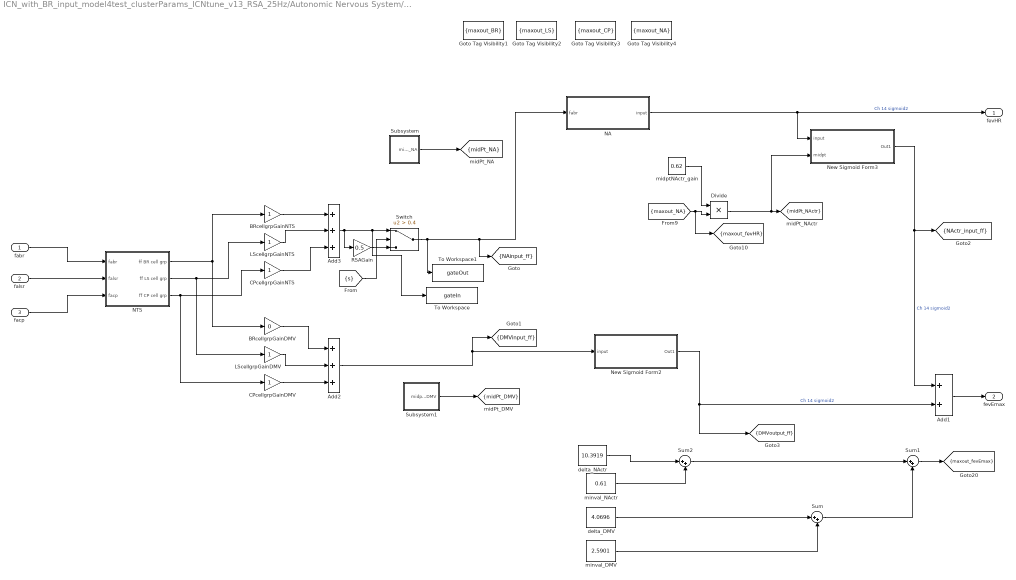
== system ICN_with_BR_input_model4test_clusterParams_ICNtune_v13_RSA_25Hz/Autonomic Nervous System/Brainstem Vagal efferents  ==
  fabr : Inport
  falsr : Inport  Port=2
  facp : Inport  Port=3
  Add1 : Sum
  Add2 : Sum  Inputs=+++
  Add3 : Sum  Inputs=+++
  BRcellgrpGainDMV : Gain  Gain=0
  BRcellgrpGainNTS : Gain
  CPcellgrpGainDMV : Gain
  CPcellgrpGainNTS : Gain
  Divide : Product  Inputs=**
  Goto Tag Visibility1 : GotoTagVisibility  GotoTag=maxout_BR
  Goto Tag Visibility2 : GotoTagVisibility  GotoTag=maxout_LS
  Goto Tag Visibility3 : GotoTagVisibility  GotoTag=maxout_CP
  Goto Tag Visibility4 : GotoTagVisibility  GotoTag=maxout_NA
  LScellgrpGainDMV : Gain
  LScellgrpGainNTS : Gain
  NA : Subsystem
  NTS : Subsystem
  New Sigmoid Form2 : Subsystem
  New Sigmoid Form3 : Subsystem
  RSAGain : Gain  Gain=0.5
  Subsystem : Subsystem
  Subsystem1 : Subsystem
  Sum : Sum  Inputs=|++
  Sum1 : Sum  Inputs=|++
  Sum2 : Sum  Inputs=|++
  Switch : Switch  Criteria=u2 > Threshold  Threshold=0.4
  To Workspace : ToWorkspace  VariableName=gateIn  SampleTime=-1
  To Workspace1 : ToWorkspace  VariableName=gateOut  SampleTime=-1
  delta_DMV : Constant  Value=4.0696
  delta_NActr : Constant  Value=10.3919
  midptNActr_gain : Constant  Value=0.62
  minval_DMV : Constant  Value=2.5901
  minval_NActr : Constant  Value=0.61
  fevHR : Outport
  fevEmax : Outport  Port=2
  tag scope: DMVinput_ff=scoped, DMVoutput_ff=scoped, NActr_input_ff=scoped, NAinput_ff=scoped, maxout_fevEmax=scoped, maxout_fevHR=scoped, midPt_DMV=scoped, midPt_NA=scoped, midPt_NActr=scoped
  wires:
  facp/1 -> NTS/3(facp)
  fabr/1 -> NTS/1(fabr)
  Add1/1 -> fevEmax/1
  NTS/1(ff BR cell grp) -> BRcellgrpGainDMV/1, BRcellgrpGainNTS/1
  NTS/2(ff LS cell grp) -> LScellgrpGainNTS/1, LScellgrpGainDMV/1
  NTS/3(ff CP cell grp) -> CPcellgrpGainNTS/1, CPcellgrpGainDMV/1
  BRcellgrpGainNTS/1 -> Add3/1
  CPcellgrpGainNTS/1 -> Add3/3
  BRcellgrpGainDMV/1 -> Add2/1
  CPcellgrpGainDMV/1 -> Add2/3
  minval_NActr/1 -> Sum2/2
  delta_NActr/1 -> Sum2/1
  minval_DMV/1 -> Sum/2
  delta_DMV/1 -> Sum/1
  falsr/1 -> NTS/2(falsr)
  [maxout_NA] -> [maxout_fevHR], Divide/2
  LScellgrpGainNTS/1 -> Add3/2
  LScellgrpGainDMV/1 -> Add2/2
  Add2/1 -> New Sigmoid Form2/1(input), [DMVinput_ff]
  Subsystem1/1(midpt_DMV) -> [midPt_DMV]
  Subsystem/1(midpt_NA) -> [midPt_NA]
  Divide/1 -> [midPt_NActr], New Sigmoid Form3/2(midpt)
  midptNActr_gain/1 -> Divide/1
  Sum/1 -> Sum1/2
  Sum2/1 -> Sum1/1
  Sum1/1 -> [maxout_fevEmax]
  NA/1(input) -> New Sigmoid Form3/1(input), fevHR/1  "Ch 14 sigmoid2"
  New Sigmoid Form3/1(Out1) -> Add1/1, [NActr_input_ff]  "Ch 14 sigmoid2"
  New Sigmoid Form2/1(Out1) -> Add1/2, [DMVoutput_ff]  "Ch 14 sigmoid2"
  Add3/1 -> To Workspace/1, Switch/1, RSAGain/1
  RSAGain/1 -> Switch/3
  [s] -> Switch/2
  Switch/1 -> To Workspace1/1, NA/1(fabr), [NAinput_ff]

== system ICN_with_BR_input_model4test_clusterParams_ICNtune_v13_RSA_25Hz/Autonomic Nervous System/Cardiopulmonary Baroreceptors ==
  Ptrans : Inport
  " 1/[taul 1]" : TransferFcn  Denominator=[2 1]
  Constant3 : Constant
  Divide : Product  Inputs=*/
  Divide1 : Product  Inputs=*/
  Exp : Math  SaturateOnIntegerOverflow=on
  Ptn : Constant  Value=10.8
  Sum : Sum  Inputs=|+-
  Sum1 : Sum  Inputs=|++
  fmaxl : Constant  Value=20
  kl : Constant  Value=1.4286
  facp : Outport
  wires:
  " 1/[taul 1]"/1 -> Sum/2
  Ptrans/1 -> " 1/[taul 1]"/1
  fmaxl/1 -> Divide/1
  Ptn/1 -> Sum/1
  Sum/1 -> Divide1/1
  kl/1 -> Divide1/2
  Divide1/1 -> Exp/1
  Exp/1 -> Sum1/1
  Constant3/1 -> Sum1/2
  Sum1/1 -> Divide/2
  Divide/1 -> facp/1

== system ICN_with_BR_input_model4test_clusterParams_ICNtune_v13_RSA_25Hz/Autonomic Nervous System/Carotid Sinus (baroreceptors) ==
  Pin : Inport
  (tauz 1) (taup 1) : TransferFcn  Numerator=[6.37 1]  Denominator=[2.076 1]
  Constant3 : Constant  Value=11.758
  Constant4 : Constant
  Divide : Product  Inputs=*/
  Divide1 : Product  Inputs=*/
  Divide2 : Product  Inputs=**
  Exp : Math  SaturateOnIntegerOverflow=on
  Pn : Constant  Value=92
  Sum : Sum  Inputs=|-+
  Sum1 : Sum  Inputs=|++
  Sum2 : Sum  Inputs=|++
  fmax : Constant  Value=47.78
  fmin : Constant  Value=2.52
  fabr : Outport
  tag scope: maxout_fabr=scoped
  wires:
  (tauz 1) (taup 1)/1 -> Sum/2
  Pin/1 -> (tauz 1) (taup 1)/1
  Pn/1 -> Sum/1
  Constant3/1 -> Divide/2
  Sum/1 -> Divide/1
  Divide/1 -> Exp/1
  Exp/1 -> Divide2/2, Sum1/1
  Constant4/1 -> Sum1/2
  fmax/1 -> [maxout_fabr], Divide2/1
  Divide2/1 -> Sum2/1
  fmin/1 -> Sum2/2
  Sum2/1 -> Divide1/1
  Sum1/1 -> Divide1/2
  Divide1/1 -> fabr/1

== system ICN_with_BR_input_model4test_clusterParams_ICNtune_v13_RSA_25Hz/Autonomic Nervous System/Emaxlv_inv ==
  fev : Inport
  fes : Inport  Port=2
  Add1 : Sum  Inputs=+++
  Add2 : Sum
  Clock : Clock
  Emaxlv0_denervated (Emaxlv0) : Constant  Value=0.25659999999999994
  Emaxlv_symp : Subsystem
  Emaxlv_vag : Subsystem
  Math Function7 : Math  Operator=reciprocal  SignedPower=on  SaturateOnIntegerOverflow=on
  Pcs_start : Constant
  Scope6 : Scope
  const : Constant  Value=0
  tstall : Switch  Criteria=u2 > Threshold  Threshold=1
  Emaxlv : Outport
  wires:
  Emaxlv_symp/1(1/Emaxlv) -> Scope6/1, Add1/2
  Math Function7/1 -> Add2/1
  Emaxlv_vag/1(1/Emaxlv) -> Add1/1
  Emaxlv0_denervated (Emaxlv0)/1 -> Add2/2
  const/1 -> Add1/3
  Clock/1 -> tstall/2
  Pcs_start/1 -> tstall/3
  tstall/1 -> Math Function7/1
  Add1/1 -> tstall/1
  fes/1 -> Emaxlv_symp/1(fes)
  fev/1 -> Emaxlv_vag/1(fev)
  Add2/1 -> Emaxlv/1

== system ICN_with_BR_input_model4test_clusterParams_ICNtune_v13_RSA_25Hz/Autonomic Nervous System/Emaxrv_inv ==
  fev : Inport
  fes : Inport  Port=2
  Add3 : Sum  Inputs=+++
  Add4 : Sum
  Clock2 : Clock
  Emaxlv0_denervated1 : Constant  Value=1.283*0.5903
  Emaxlv_symp1 : Subsystem
  Emaxlv_vag1 : Subsystem
  Math Function2 : Math  Operator=reciprocal  SignedPower=on  SaturateOnIntegerOverflow=on
  Pcs_start2 : Constant
  Switch2 : Switch  Criteria=u2 > Threshold  Threshold=1
  const1 : Constant  Value=0
  Emaxrv : Outport
  wires:
  Switch2/1 -> Math Function2/1
  Clock2/1 -> Switch2/2
  Add3/1 -> Switch2/1
  Emaxlv_symp1/1(1/Emarlv) -> Add3/2
  Math Function2/1 -> Add4/1
  const1/1 -> Add3/3
  Emaxlv0_denervated1/1 -> Add4/2
  Pcs_start2/1 -> Switch2/3
  Emaxlv_vag1/1(1/Emaxrv) -> Add3/1
  fev/1 -> Emaxlv_vag1/1(fev)
  fes/1 -> Emaxlv_symp1/1(fes)
  Add4/1 -> Emaxrv/1
